simulink model "parrot_gettingstarted"  (R2022a)
settings: Solver=FixedStepAuto  StartTime=0.0  StopTime=100  RelTol=1e-3
InitFcn:
  | load('BusDefinitions.mat')
values from neighbouring files (symbols this model uses):
  all_cov = [0.000210145415622 5.90055533394e-05 -6.5320482463e-06 7.16185822967e-05 0.000233478946029 1.6317851987e-05 7.07877552486e-06 -4.63849255539e-06 -1.33013045343e-05 -0.0012667349074 5.90055533394e-05 0.0112626235932 ... (100 elements, 10x10)]    [cov_data.mat]
  ff = 1.1    [Linearize_Fast.m]
  g = 9.81    [Linearize_Fast.m]    (also in Param_set.m = 9.8)
  ground_alt = 180.2070    (= 180.207)    [Linearize_Fast.m]
  m = 0.068    [Param_set.m]
  Mixer = double(subs(n_lin, [u_vec; a; b; c; d;], [.66708; 0; 0; 0;(1.86e-6);(8.856e-8);(8.856e-8);(9.766e-9)]))    [Linearize_Fast.m]
undefined symbols (not defined in the file or in its folder): codertarget, Discrete, K_PD, K_psi, K_u, K_v, Time
libraries: ctrlSharedLib x5
settings Model: ExtModeTrigDuration=80  Creator=The MathWorks, Inc.  LastModifiedBy=Willi
settings SolverCC: AlgebraicLoopSolver=TrustRegion
settings DataIOCC: ReturnWorkspaceOutputs=off
settings OptimizationCC: PassReuseOutputArgsThreshold=0  MaxStackSize=64
settings DebuggingCC: ParameterTunabilityLossMsg=error  UnconnectedInputMsg=warning  UnconnectedOutputMsg=warning  UnconnectedLineMsg=warning  PregeneratedLibrarySubsystemCodeDiagnostic=none  SFMachineParentedDataDiag=warning  ArithmeticOperatorsInVariantConditions=warning
settings HardwareCC: ProdBitPerPointer=32  ProdBitPerSizeT=32  ProdBitPerPtrDiffT=32  ProdLargestAtomicInteger=Long  ProdWordSize=32  ProdHWDeviceType=ARM Compatible->ARM 9  UseEmbeddedCoderFeatures=off
settings SFSimCC: SimUseLocalCustomCode=off  MATLABDynamicMemAlloc=off  CustomCodeUndefinedFunction=UseInterfaceOnly
settings RTWCC: SystemTargetFile=ert.tlc  HardwareBoard=PARROT Mambo  TemplateMakefile=ert_default_tmf  GenerateReport=on  RTWUseLocalCustomCode=off  Toolchain=Sourcery G++ Lite GNU Toolchain for Drones  BuildConfiguration=Specify  LaunchReport=on
settings CodeAppCC: ForceParamTrailComments=on  OperatorAnnotations=on  StateflowObjectComments=on
settings ERTTargetCC: ERTCustomFileBanners=off  MatFileLogging=on  SupportContinuousTime=on  SupportNonInlinedSFcns=on  RemoveResetFunc=off  ModelStepFunctionPrototypeControlCompliant=off

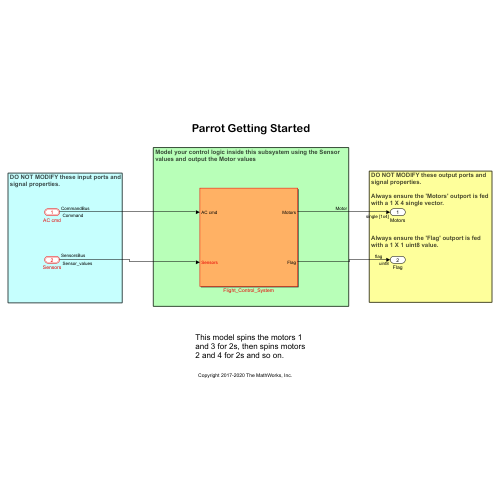
[thumbnail: Simulink's stored preview of the top-level diagram]
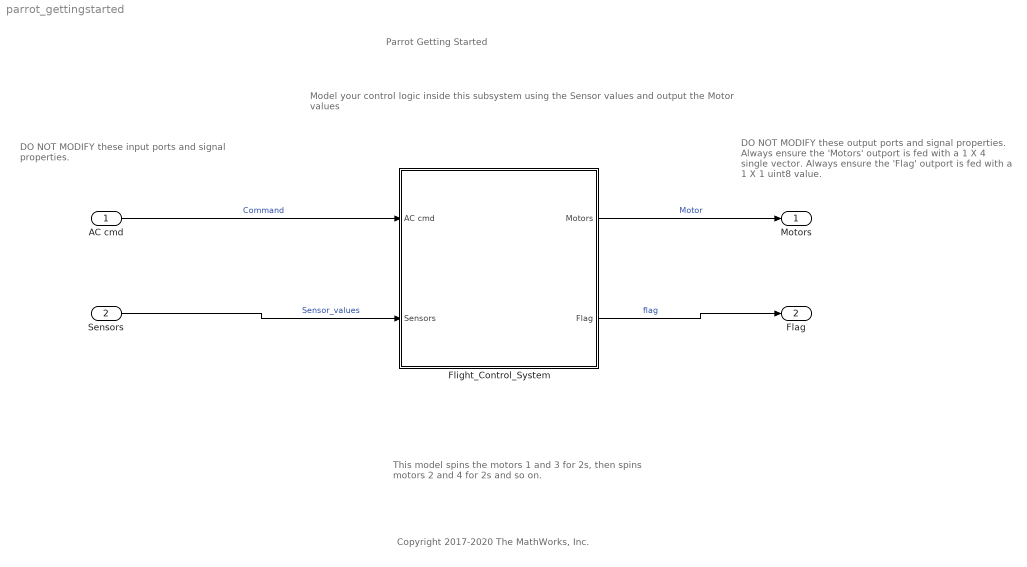
== system parrot_gettingstarted ==
  note: Model your control logic inside this subsystem using the Sensor
      | values and output the Motor values
  note: DO NOT MODIFY these output ports and
      | signal properties.
      |
      | Always ensure the 'Motors' outport is fed
      | with a 1 X 4 single vector.
      |
      |
      |
      |
      | Always ensure the 'Flag' outport is fed
      | with a 1 X 1 uint8 value.
  note: DO NOT MODIFY these input ports and
      | signal properties.
  note: This model spins the motors 1 and 3 for 2s, then spins motors 2 and 4 for 2s and so on.
  note: Copyright 2017-2020 The MathWorks, Inc.
  note: Parrot Getting Started
  AC cmd : Inport  OutDataTypeStr=Bus: CommandBus  BusOutputAsStruct=on
  Sensors : Inport  Port=2  OutDataTypeStr=Bus: SensorsBus  BusOutputAsStruct=on
  Flight_Control_System : Subsystem  InitFcn=codertarget.parrot.internal.fcsSubsystemCallback(gcb);
  Motors : Outport  OutDataTypeStr=single  PortDimensions=[1 4]  VectorParamsAs1DForOutWhenUnconnected=off
  Flag : Outport  Port=2  OutDataTypeStr=uint8  PortDimensions=1  VectorParamsAs1DForOutWhenUnconnected=off
  wires:
  Flight_Control_System/1(Motors) -> Motors/1  "Motor"
  AC cmd/1 -> Flight_Control_System/1(AC cmd)  "Command"
  Sensors/1 -> Flight_Control_System/2(Sensors)  "Sensor_values"
  Flight_Control_System/2(Flag) -> Flag/1  "flag"

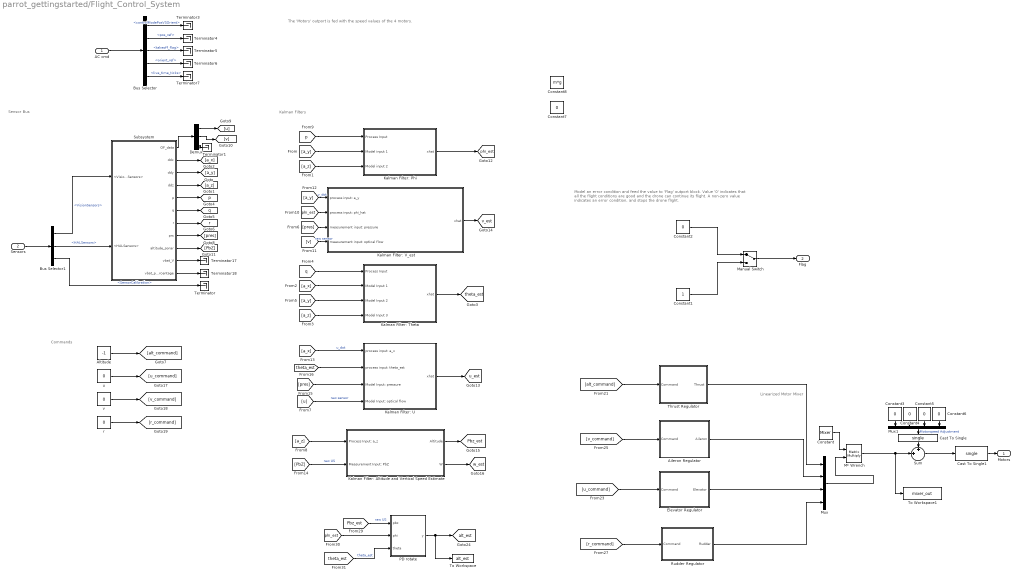
== system parrot_gettingstarted/Flight_Control_System ==
  note: Kalman Filters
  note: Sensor Bus
  note: Linearized Motor Mixer
  note: The 'Motors' outport is fed with the speed values of the 4 motors.
  note: Model an error condition and feed the value to 'Flag' outport block.
      | Value '0' indicates that all the flight conditions are good and the drone
      | can continue its flight.
      | A non-zero value indicates an error condition, and stops the drone
      | flight.
  note: Commands
  AC cmd : Inport
  Sensors : Inport  Port=2
  Aileron Regulator : Subsystem
  Altitude : Constant  Value=-1
  Bus Selector : BusSelector  OutputSignals=controlModePosVSOrient,pos_ref,takeoff_flag,orient_ref,live_time_ticks
  Bus Selector1 : BusSelector  OutputSignals=VisionSensors,HALSensors,SensorCalibration
  Cast To Single : DataTypeConversion  OutDataTypeStr=single  SaturateOnIntegerOverflow=off  RndMeth=Floor
  Cast To Single1 : DataTypeConversion  OutDataTypeStr=single  SaturateOnIntegerOverflow=off  RndMeth=Floor
  Constant : Constant  Value=Mixer
  Constant1 : Constant  OutDataTypeStr=uint8
  Constant2 : Constant  Value=0  OutDataTypeStr=uint8
  Constant{3..7} (5 alike) : Constant  Value=0
  Constant8 : Constant  Value=m*g
  Demux : Demux  Outputs=3
  Elevator Regulator : Subsystem
  Kalman Filter: Altitude and Vertical Speed Estimate : Subsystem
  Kalman Filter: Phi : Subsystem
  Kalman Filter: Theta : Subsystem
  Kalman Filter: U : Subsystem
  Kalman Filter: V_est : Subsystem
  M* Wrench : Product  Multiplication=Matrix(*)
  Manual Switch : ManualSwitch
  Mux : Mux
  Mux1 : Mux
  PD rotate : MATLAB Function  TreatAsAtomicUnit=on
  Rudder Regulator : Subsystem
  Subsystem : Subsystem
  Sum : Sum  Inputs=+|+||
  Terminator{,1,3..7,17..18} (9 alike) : Terminator
  Thrust Regulator : Subsystem
  To Workspace : ToWorkspace  VariableName=alt_est  SaveFormat=Structure With Time  SampleTime=-1
  To Workspace1 : ToWorkspace  VariableName=mixer_out  SaveFormat=Structure With Time  SampleTime=-1
  r : Constant  Value=0
  u : Constant  Value=0
  v : Constant  Value=0
  Motors : Outport  VectorParamsAs1DForOutWhenUnconnected=off
  Flag : Outport  Port=2  VectorParamsAs1DForOutWhenUnconnected=off
  tag scope: Pbz_est=global, alt_est=global, p=global, phi_est=global, q=global, r=global, theta_est=global, u_est=global, v_est=global, w_est=global
  wires:
  AC cmd/1 -> Bus Selector/1
  Bus Selector/1 -> Terminator3/1  "<controlModePosVSOrient>"
  Bus Selector/2 -> Terminator4/1  "<pos_ref>"
  Bus Selector/3 -> Terminator5/1  "<takeoff_flag>"
  Bus Selector/4 -> Terminator6/1  "<orient_ref>"
  Bus Selector/5 -> Terminator7/1  "<live_time_ticks>"
  Manual Switch/1 -> Flag/1
  Constant2/1 -> Manual Switch/1
  Constant1/1 -> Manual Switch/2
  Subsystem/11(vbat_percentage) -> Terminator18/1
  Bus Selector1/3 -> Terminator/1  "<SensorCalibration>"
  Subsystem/8(prs) -> [pres]
  Bus Selector1/2 -> Subsystem/2(<HALSensors>)  "<HALSensors>"
  Bus Selector1/1 -> Subsystem/1(<VisionSensors>)  "<VisionSensors>"
  Subsystem/1(OF_data) -> Demux/1
  Subsystem/4(ddz) -> [a_z]
  Subsystem/3(ddy) -> [a_y]
  Subsystem/9(altitude_sonar) -> [PbZ]
  Subsystem/10(vbat_V) -> Terminator17/1
  Subsystem/2(ddx) -> [a_x]
  Sensors/1 -> Bus Selector1/1
  Sum/1 -> Cast To Single1/1
  Mux1/1 -> Cast To Single/1  "Motorspeed Adjustment"
  Cast To Single/1 -> Sum/1
  Constant6/1 -> Mux1/4
  Constant5/1 -> Mux1/3
  Constant3/1 -> Mux1/1
  Constant4/1 -> Mux1/2
  Constant/1 -> M* Wrench/1
  Demux/1 -> [u]
  Demux/2 -> [v]
  Demux/3 -> Terminator1/1
  Subsystem/5(p) -> [p]
  Subsystem/6(q) -> [q]
  Subsystem/7(r) -> [r]
  [a_z] -> Kalman Filter: Phi/3(Model input 2)
  [a_y] -> Kalman Filter: Phi/2(Model input 1)
  Kalman Filter: Phi/1(xhat) -> [phi_est]
  [p] -> Kalman Filter: Phi/1(Process Input)
  [q] -> Kalman Filter: Theta/1(Process Input)
  Kalman Filter: Theta/1(xhat) -> [theta_est]
  [a_z] -> Kalman Filter: Theta/4(Model Input 3)
  [a_x] -> Kalman Filter: Theta/2(Model Input 1)
  [a_y] -> Kalman Filter: Theta/3(Model Input 2)
  [theta_est] -> Kalman Filter: U/2(process input: theta_est)
  [u] -> Kalman Filter: U/4(Model Input: optical flow)  "raw sensor"
  [a_x] -> Kalman Filter: U/1(process input: a_x)  "u_dot"
  Kalman Filter: U/1(xhat) -> [u_est]
  [pres] -> Kalman Filter: U/3(Model Input: pressure)
  [a_z] -> Kalman Filter: Altitude and Vertical Speed Estimate/1("Process Input: a_z ")
  Kalman Filter: Altitude and Vertical Speed Estimate/1(Altitude) -> [Pbz_est]
  [PbZ] -> Kalman Filter: Altitude and Vertical Speed Estimate/2(Measurement Input: PbZ)  "raw US"
  Kalman Filter: Altitude and Vertical Speed Estimate/2(W) -> [w_est]
  [a_y] -> Kalman Filter: V_est/1("process input: a_y   ")  "v_dot"
  [pres] -> Kalman Filter: V_est/3(measurement input: pressure)
  [v] -> Kalman Filter: V_est/4(measurement input: optical flow)  "raw sensor"
  Kalman Filter: V_est/1(xhat) -> [v_est]
  [phi_est] -> Kalman Filter: V_est/2("process input: phi_hat ")
  [theta_est] -> PD rotate/3(theta)  "theta_est"
  PD rotate/1(y) -> To Workspace/1, [alt_est]
  [Pbz_est] -> PD rotate/1(pbz)  "raw US"
  [phi_est] -> PD rotate/2(phi)
  r/1 -> [r_command]
  v/1 -> [v_command]
  u/1 -> [u_command]
  Altitude/1 -> [alt_command]
  [alt_command] -> Thrust Regulator/1(Command)
  Mux/1 -> M* Wrench/2
  Cast To Single1/1 -> Motors/1
  M* Wrench/1 -> Sum/2, To Workspace1/1
  [r_command] -> Rudder Regulator/1(Command)
  [u_command] -> Elevator Regulator/1(Command)
  [v_command] -> Aileron Regulator/1(Command)
  Rudder Regulator/1(Rudder) -> Mux/4
  Thrust Regulator/1(Thrust) -> Mux/1
  Elevator Regulator/1(Elevator) -> Mux/3
  Aileron Regulator/1(Aileron) -> Mux/2

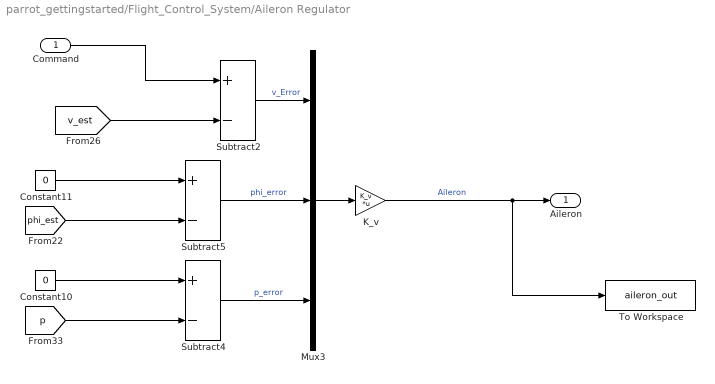
== system parrot_gettingstarted/Flight_Control_System/Aileron Regulator ==
  Command : Inport
  Constant10 : Constant  Value=0
  Constant11 : Constant  Value=0
  K_v : Gain  Gain=K_v  Multiplication=Matrix(K*u)
  Mux3 : Mux  Inputs=3
  Subtract2 : Sum  Inputs=+-
  Subtract4 : Sum  Inputs=+-
  Subtract5 : Sum  Inputs=+-
  To Workspace : ToWorkspace  VariableName=aileron_out  SaveFormat=Timeseries  SampleTime=-1
  Aileron : Outport
  wires:
  [p] -> Subtract4/2
  [v_est] -> Subtract2/2
  Constant11/1 -> Subtract5/1
  [phi_est] -> Subtract5/2
  Subtract5/1 -> Mux3/2  "phi_error"
  Subtract2/1 -> Mux3/1  "v_Error"
  Mux3/1 -> K_v/1
  Subtract4/1 -> Mux3/3  "p_error"
  Constant10/1 -> Subtract4/1
  K_v/1 -> To Workspace/1, Aileron/1  "Aileron"
  Command/1 -> Subtract2/1

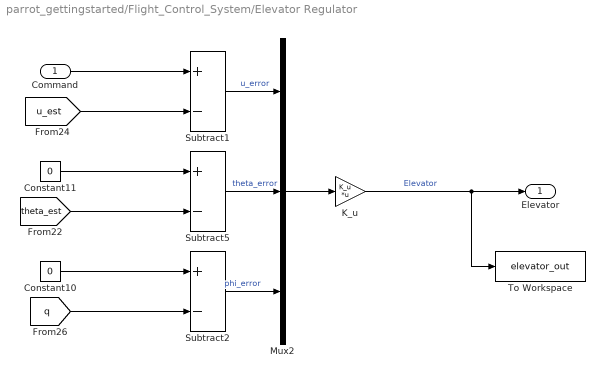
== system parrot_gettingstarted/Flight_Control_System/Elevator Regulator ==
  Command : Inport
  Constant10 : Constant  Value=0
  Constant11 : Constant  Value=0
  K_u : Gain  Gain=K_u  Multiplication=Matrix(K*u)
  Mux2 : Mux  Inputs=3
  Subtract1 : Sum  Inputs=+-
  Subtract2 : Sum  Inputs=+-
  Subtract5 : Sum  Inputs=+-
  To Workspace : ToWorkspace  VariableName=elevator_out  SaveFormat=Timeseries  SampleTime=-1
  Elevator : Outport
  wires:
  [theta_est] -> Subtract5/2
  [u_est] -> Subtract1/2
  Constant10/1 -> Subtract2/1
  Constant11/1 -> Subtract5/1
  Subtract5/1 -> Mux2/2  "theta_error"
  Subtract1/1 -> Mux2/1  "u_error"
  Subtract2/1 -> Mux2/3  "phi_error"
  Mux2/1 -> K_u/1
  [q] -> Subtract2/2
  K_u/1 -> To Workspace/1, Elevator/1  "Elevator"
  Command/1 -> Subtract1/1

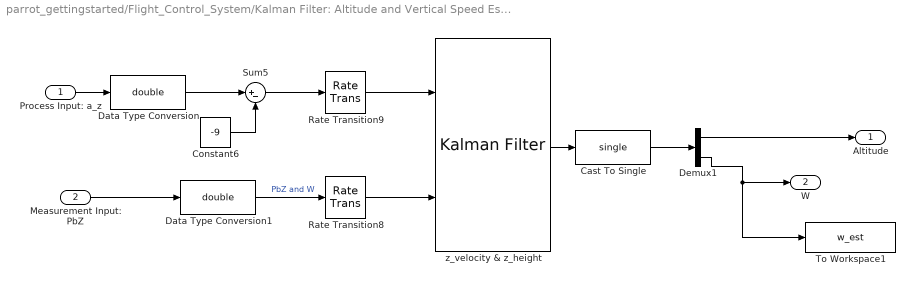
== system parrot_gettingstarted/Flight_Control_System/Kalman Filter: Altitude and Vertical Speed Estimate ==
  "Process Input: a_z " : Inport
  Measurement Input: PbZ : Inport  Port=2
  Cast To Single : DataTypeConversion  OutDataTypeStr=single  SaturateOnIntegerOverflow=off  RndMeth=Floor
  Constant6 : Constant  Value=-9
  Data Type Conversion : DataTypeConversion  OutDataTypeStr=double  SaturateOnIntegerOverflow=off  RndMeth=Floor
  Data Type Conversion1 : DataTypeConversion  OutDataTypeStr=double  SaturateOnIntegerOverflow=off  RndMeth=Floor
  Demux1 : Demux  Outputs=2
  Rate Transition8 : RateTransition  OutPortSampleTime=1/200
  Rate Transition9 : RateTransition  OutPortSampleTime=1/200
  Sum5 : Sum  Inputs=|+-
  To Workspace1 : ToWorkspace  VariableName=w_est  SaveFormat=Structure With Time  SampleTime=-1
  z_velocity & z_height : ctrlSharedLib/Kalman Filter  TimeDomain=Discrete-Time  UseCurrentEstimator=on  ModelSource=Individual A, B, C, D matrices  ModelSourceVariable=ss(0.95,1,1,0,1)  A=[1 1/200;0 1]  B=[0; 1/200]  C=[1 0]  D=0  NumberOfStates=1  NumberOfInputs=1  NumberOfOutputs=1  InitialEstimateSource=Dialog  X0=0  P0=10  UseK=off  UseGH=off  NumberOfProcessNoiseInputs=1  G=1  TimeInvariantG=on  H=0  TimeInvariantH=on  Q=all_cov(7,7)/1000  TimeInvariantQ=on  R=all_cov(1,1)*50  TimeInvariantR=on  N=0  TimeInvariantN=on  AddInputPort=on  AddEnablePort=off  OutputEstimatedY=off  OutputP=off  Ts=-1
  Altitude : Outport
  W : Outport  Port=2
  wires:
  Data Type Conversion1/1 -> Rate Transition8/1  "PbZ and W"
  Constant6/1 -> Sum5/2
  Demux1/1 -> Altitude/1
  z_velocity & z_height/1 -> Cast To Single/1
  Sum5/1 -> Rate Transition9/1
  Data Type Conversion/1 -> Sum5/1
  Rate Transition9/1 -> z_velocity & z_height/1
  Rate Transition8/1 -> z_velocity & z_height/2
  Measurement Input: PbZ/1 -> Data Type Conversion1/1
  Demux1/2 -> W/1, To Workspace1/1
  "Process Input: a_z "/1 -> Data Type Conversion/1
  Cast To Single/1 -> Demux1/1

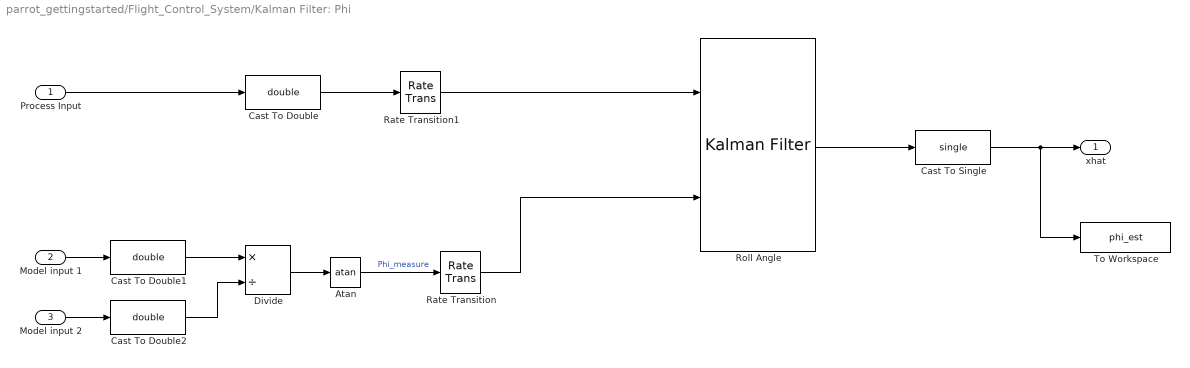
== system parrot_gettingstarted/Flight_Control_System/Kalman Filter: Phi ==
  Process Input : Inport
  Model input 1 : Inport  Port=2
  Model input 2 : Inport  Port=3
  Atan : Trigonometry  Operator=atan
  Cast To Double : DataTypeConversion  OutDataTypeStr=double  SaturateOnIntegerOverflow=off  RndMeth=Floor
  Cast To Double1 : DataTypeConversion  OutDataTypeStr=double  SaturateOnIntegerOverflow=off  RndMeth=Floor
  Cast To Double2 : DataTypeConversion  OutDataTypeStr=double  SaturateOnIntegerOverflow=off  RndMeth=Floor
  Cast To Single : DataTypeConversion  OutMax=1  OutDataTypeStr=single  SaturateOnIntegerOverflow=off  RndMeth=Floor
  Divide : Product  Inputs=*/
  Rate Transition : RateTransition  OutPortSampleTime=1/200
  Rate Transition1 : RateTransition  OutPortSampleTime=1/200
  Roll Angle : ctrlSharedLib/Kalman Filter  TimeDomain=Discrete-Time  UseCurrentEstimator=on  ModelSource=Individual A, B, C, D matrices  ModelSourceVariable=ss(0.95,1,1,0,1)  A=[1]  B=[1/200]  C=[1]  D=0  NumberOfStates=1  NumberOfInputs=1  NumberOfOutputs=1  InitialEstimateSource=Dialog  X0=0  P0=10  UseK=off  UseGH=off  NumberOfProcessNoiseInputs=1  G=1  TimeInvariantG=on  H=0  TimeInvariantH=on  Q=.0133/200  TimeInvariantQ=on  R=.0101  TimeInvariantR=on  N=0  TimeInvariantN=on  AddInputPort=on  AddEnablePort=off  OutputEstimatedY=off  OutputP=off  Ts=-1
  To Workspace : ToWorkspace  VariableName=phi_est  SaveFormat=Structure With Time  SampleTime=-1
  xhat : Outport
  wires:
  Divide/1 -> Atan/1
  Atan/1 -> Rate Transition/1  "Phi_measure"
  Process Input/1 -> Cast To Double/1
  Rate Transition/1 -> Roll Angle/2
  Rate Transition1/1 -> Roll Angle/1
  Cast To Double/1 -> Rate Transition1/1
  Cast To Double1/1 -> Divide/1
  Model input 1/1 -> Cast To Double1/1
  Model input 2/1 -> Cast To Double2/1
  Cast To Double2/1 -> Divide/2
  Cast To Single/1 -> To Workspace/1, xhat/1
  Roll Angle/1 -> Cast To Single/1

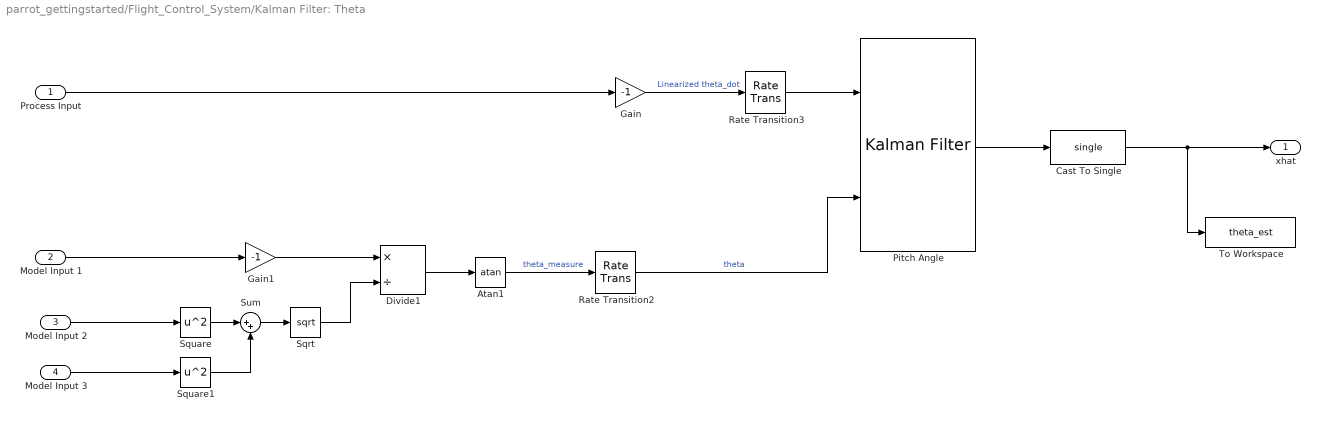
== system parrot_gettingstarted/Flight_Control_System/Kalman Filter: Theta ==
  Process Input : Inport
  Model Input 1 : Inport  Port=2
  Model Input 2 : Inport  Port=3
  Model Input 3 : Inport  Port=4
  Atan1 : Trigonometry  Operator=atan
  Cast To Single : DataTypeConversion  OutDataTypeStr=single  SaturateOnIntegerOverflow=off  RndMeth=Floor
  Divide1 : Product  Inputs=*/
  Gain : Gain  Gain=-1
  Gain1 : Gain  Gain=-1
  Pitch Angle : ctrlSharedLib/Kalman Filter  TimeDomain=Discrete-Time  UseCurrentEstimator=on  ModelSource=Individual A, B, C, D matrices  ModelSourceVariable=ss(0.95,1,1,0,1)  A=[1]  B=[1/200]  C=[1]  D=0  NumberOfStates=1  NumberOfInputs=1  NumberOfOutputs=1  InitialEstimateSource=Dialog  X0=0  P0=10  UseK=off  UseGH=off  NumberOfProcessNoiseInputs=1  G=1  TimeInvariantG=on  H=0  TimeInvariantH=on  Q=.0085/1000  TimeInvariantQ=on  R=.0066/10  TimeInvariantR=on  N=0  TimeInvariantN=on  AddInputPort=on  AddEnablePort=off  OutputEstimatedY=off  OutputP=off  Ts=-1
  Rate Transition2 : RateTransition  OutPortSampleTime=1/200
  Rate Transition3 : RateTransition  OutPortSampleTime=1/200
  Sqrt : Sqrt
  Square : Math  Operator=square
  Square1 : Math  Operator=square
  Sum : Sum  Inputs=|++
  To Workspace : ToWorkspace  VariableName=theta_est  SaveFormat=Structure With Time  SampleTime=-1
  xhat : Outport
  wires:
  Gain1/1 -> Divide1/1
  Divide1/1 -> Atan1/1
  Model Input 2/1 -> Square/1
  Rate Transition3/1 -> Pitch Angle/1
  Sum/1 -> Sqrt/1
  Square/1 -> Sum/1
  Square1/1 -> Sum/2
  Atan1/1 -> Rate Transition2/1  "theta_measure"
  Sqrt/1 -> Divide1/2
  Rate Transition2/1 -> Pitch Angle/2  "theta"
  Gain/1 -> Rate Transition3/1  "Linearized theta_dot"
  Process Input/1 -> Gain/1
  Model Input 1/1 -> Gain1/1
  Model Input 3/1 -> Square1/1
  Cast To Single/1 -> xhat/1, To Workspace/1
  Pitch Angle/1 -> Cast To Single/1

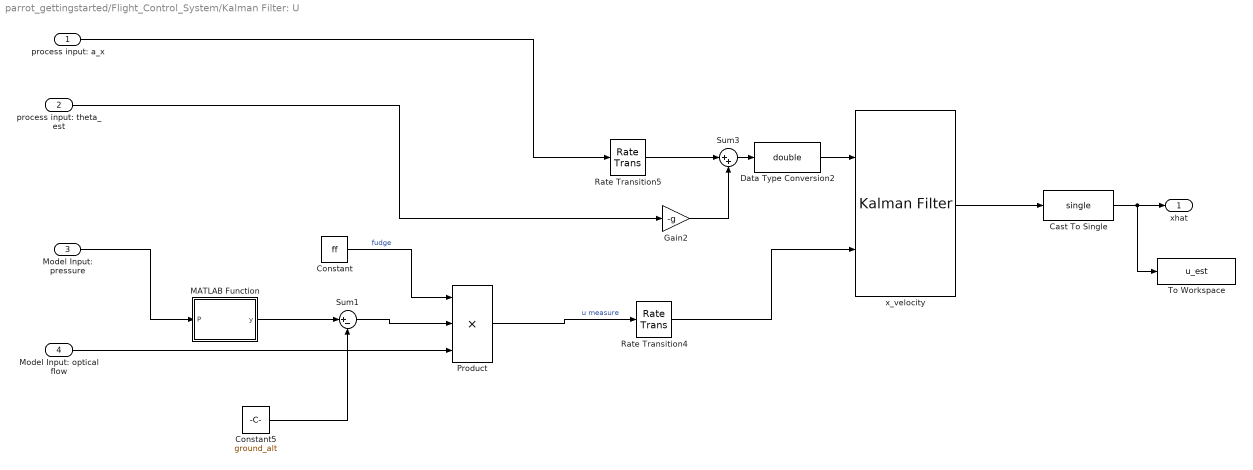
== system parrot_gettingstarted/Flight_Control_System/Kalman Filter: U ==
  process input: a_x : Inport
  process input: theta_est : Inport  Port=2
  Model Input: pressure : Inport  Port=3
  Model Input: optical flow : Inport  Port=4
  Cast To Single : DataTypeConversion  OutDataTypeStr=single  SaturateOnIntegerOverflow=off  RndMeth=Floor
  Constant : Constant  Value=ff
  Constant5 : Constant  Value=ground_alt
  Data Type Conversion2 : DataTypeConversion  OutDataTypeStr=double  SaturateOnIntegerOverflow=off  RndMeth=Floor
  Gain2 : Gain  Gain=-g
  MATLAB Function : MATLAB Function  TreatAsAtomicUnit=on
  Product : Product  Inputs=3
  Rate Transition4 : RateTransition  OutPortSampleTime=1/200
  Rate Transition5 : RateTransition  OutPortSampleTime=1/200
  Sum1 : Sum  Inputs=|+-
  Sum3 : Sum  Inputs=|++
  To Workspace : ToWorkspace  VariableName=u_est  SaveFormat=Structure With Time  SampleTime=-1
  x_velocity : ctrlSharedLib/Kalman Filter  TimeDomain=Discrete-Time  UseCurrentEstimator=on  ModelSource=Individual A, B, C, D matrices  ModelSourceVariable=ss(0.95,1,1,0,1)  A=[1]  B=[1/200]  C=[1]  D=0  NumberOfStates=1  NumberOfInputs=1  NumberOfOutputs=1  InitialEstimateSource=Dialog  X0=0  P0=10  UseK=off  UseGH=off  NumberOfProcessNoiseInputs=1  G=1  TimeInvariantG=on  H=0  TimeInvariantH=on  Q=.0059/200  TimeInvariantQ=on  R=all_cov(10,8)*20  TimeInvariantR=on  N=0  TimeInvariantN=on  AddInputPort=on  AddEnablePort=off  OutputEstimatedY=off  OutputP=off  Ts=-1
  xhat : Outport
  wires:
  process input: theta_est/1 -> Gain2/1
  MATLAB Function/1(y) -> Sum1/1
  Gain2/1 -> Sum3/2
  Product/1 -> Rate Transition4/1  "u measure"
  Rate Transition4/1 -> x_velocity/2
  process input: a_x/1 -> Rate Transition5/1
  Rate Transition5/1 -> Sum3/1
  Sum1/1 -> Product/2
  Data Type Conversion2/1 -> x_velocity/1
  Constant/1 -> Product/1  "fudge"
  Sum3/1 -> Data Type Conversion2/1
  Constant5/1 -> Sum1/2
  Model Input: pressure/1 -> MATLAB Function/1(P)
  Model Input: optical flow/1 -> Product/3
  Cast To Single/1 -> To Workspace/1, xhat/1
  x_velocity/1 -> Cast To Single/1

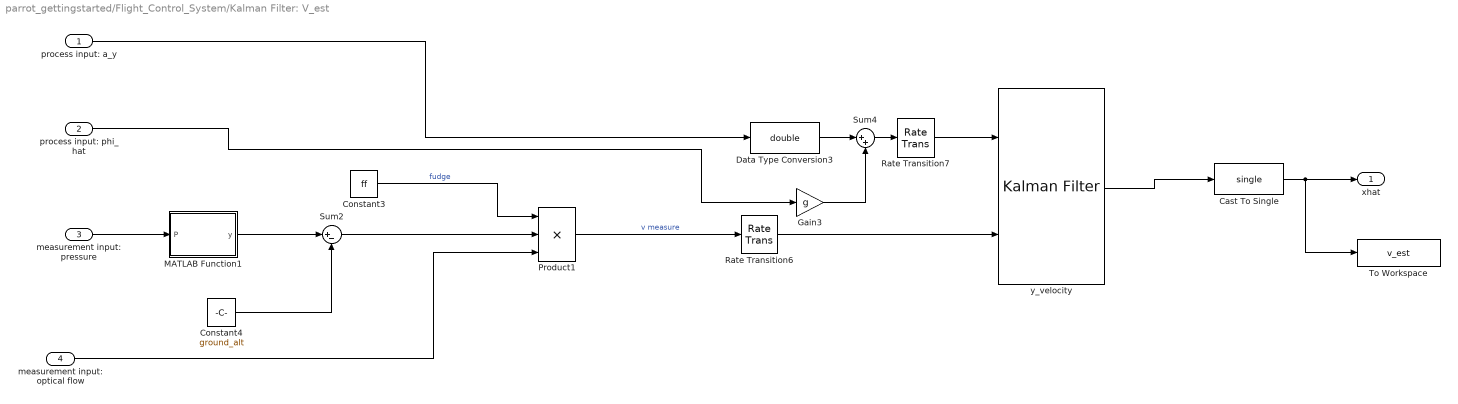
== system parrot_gettingstarted/Flight_Control_System/Kalman Filter: V_est ==
  "process input: a_y   " : Inport
  "process input: phi_hat " : Inport  Port=2
  measurement input: pressure : Inport  Port=3
  measurement input: optical flow : Inport  Port=4
  Cast To Single : DataTypeConversion  OutDataTypeStr=single  SaturateOnIntegerOverflow=off  RndMeth=Floor
  Constant3 : Constant  Value=ff
  Constant4 : Constant  Value=ground_alt
  Data Type Conversion3 : DataTypeConversion  OutDataTypeStr=double  SaturateOnIntegerOverflow=off  RndMeth=Floor
  Gain3 : Gain  Gain=g
  MATLAB Function1 : MATLAB Function  TreatAsAtomicUnit=on
  Product1 : Product  Inputs=3
  Rate Transition6 : RateTransition  OutPortSampleTime=1/200
  Rate Transition7 : RateTransition  OutPortSampleTime=1/200
  Sum2 : Sum  Inputs=|+-
  Sum4 : Sum  Inputs=|++
  To Workspace : ToWorkspace  VariableName=v_est  SaveFormat=Structure With Time  SampleTime=-1
  y_velocity : ctrlSharedLib/Kalman Filter  TimeDomain=Discrete-Time  UseCurrentEstimator=on  ModelSource=Individual A, B, C, D matrices  ModelSourceVariable=ss(0.95,1,1,0,1)  A=[1]  B=[1/200]  C=[1]  D=0  NumberOfStates=1  NumberOfInputs=1  NumberOfOutputs=1  InitialEstimateSource=Dialog  X0=0  P0=10  UseK=off  UseGH=off  NumberOfProcessNoiseInputs=1  G=1  TimeInvariantG=on  H=0  TimeInvariantH=on  Q=.0087/200  TimeInvariantQ=on  R=2.5  TimeInvariantR=on  N=0  TimeInvariantN=on  AddInputPort=on  AddEnablePort=off  OutputEstimatedY=off  OutputP=off  Ts=-1
  xhat : Outport
  wires:
  MATLAB Function1/1(y) -> Sum2/1
  Gain3/1 -> Sum4/2
  Sum2/1 -> Product1/2
  measurement input: optical flow/1 -> Product1/3
  Constant4/1 -> Sum2/2
  Product1/1 -> Rate Transition6/1  "v measure"
  Rate Transition6/1 -> y_velocity/2
  Sum4/1 -> Rate Transition7/1
  Constant3/1 -> Product1/1  "fudge"
  Rate Transition7/1 -> y_velocity/1
  Data Type Conversion3/1 -> Sum4/1
  "process input: phi_hat "/1 -> Gain3/1
  measurement input: pressure/1 -> MATLAB Function1/1(P)
  "process input: a_y   "/1 -> Data Type Conversion3/1
  Cast To Single/1 -> To Workspace/1, xhat/1
  y_velocity/1 -> Cast To Single/1

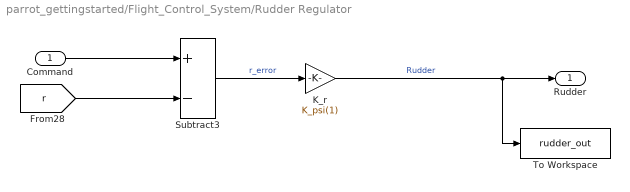
== system parrot_gettingstarted/Flight_Control_System/Rudder Regulator ==
  Command : Inport
  K_r : Gain  Gain=K_psi(1)
  Subtract3 : Sum  Inputs=+-
  To Workspace : ToWorkspace  VariableName=rudder_out  SaveFormat=Timeseries  SampleTime=-1
  Rudder : Outport
  wires:
  Subtract3/1 -> K_r/1  "r_error"
  K_r/1 -> To Workspace/1, Rudder/1  "Rudder"
  [r] -> Subtract3/2
  Command/1 -> Subtract3/1

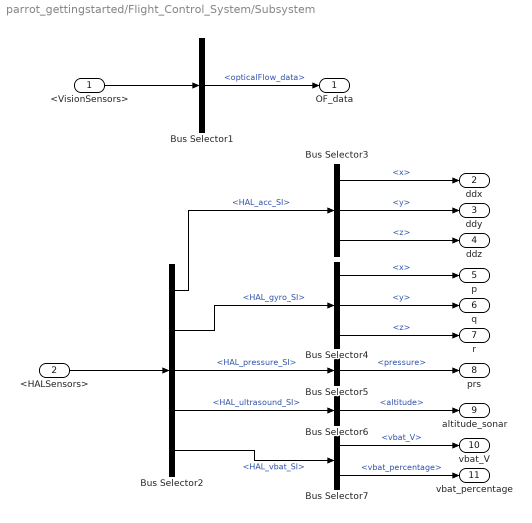
== system parrot_gettingstarted/Flight_Control_System/Subsystem ==
  <VisionSensors> : Inport
  <HALSensors> : Inport  Port=2
  Bus Selector1 : BusSelector  OutputSignals=opticalFlow_data
  Bus Selector2 : BusSelector  OutputSignals=HAL_acc_SI,HAL_gyro_SI,HAL_pressure_SI,HAL_ultrasound_SI,HAL_vbat_SI
  Bus Selector3 : BusSelector  OutputSignals=x,y,z
  Bus Selector4 : BusSelector  OutputSignals=x,y,z
  Bus Selector5 : BusSelector  OutputSignals=pressure
  Bus Selector6 : BusSelector  OutputSignals=altitude
  Bus Selector7 : BusSelector  OutputSignals=vbat_V,vbat_percentage
  OF_data : Outport  VectorParamsAs1DForOutWhenUnconnected=off
  ddx : Outport  Port=2  VectorParamsAs1DForOutWhenUnconnected=off
  ddy : Outport  Port=3  VectorParamsAs1DForOutWhenUnconnected=off
  ddz : Outport  Port=4  VectorParamsAs1DForOutWhenUnconnected=off
  p : Outport  Port=5  VectorParamsAs1DForOutWhenUnconnected=off
  q : Outport  Port=6  VectorParamsAs1DForOutWhenUnconnected=off
  r : Outport  Port=7  VectorParamsAs1DForOutWhenUnconnected=off
  prs : Outport  Port=8  VectorParamsAs1DForOutWhenUnconnected=off
  altitude_sonar : Outport  Port=9  VectorParamsAs1DForOutWhenUnconnected=off
  vbat_V : Outport  Port=10  VectorParamsAs1DForOutWhenUnconnected=off
  vbat_percentage : Outport  Port=11  VectorParamsAs1DForOutWhenUnconnected=off
  wires:
  <VisionSensors>/1 -> Bus Selector1/1
  <HALSensors>/1 -> Bus Selector2/1
  Bus Selector1/1 -> OF_data/1  "<opticalFlow_data>"
  Bus Selector2/1 -> Bus Selector3/1  "<HAL_acc_SI>"
  Bus Selector2/2 -> Bus Selector4/1  "<HAL_gyro_SI>"
  Bus Selector2/3 -> Bus Selector5/1  "<HAL_pressure_SI>"
  Bus Selector2/4 -> Bus Selector6/1  "<HAL_ultrasound_SI>"
  Bus Selector2/5 -> Bus Selector7/1  "<HAL_vbat_SI>"
  Bus Selector3/1 -> ddx/1  "<x>"
  Bus Selector3/2 -> ddy/1  "<y>"
  Bus Selector3/3 -> ddz/1  "<z>"
  Bus Selector4/2 -> q/1  "<y>"
  Bus Selector4/1 -> p/1  "<x>"
  Bus Selector4/3 -> r/1  "<z>"
  Bus Selector5/1 -> prs/1  "<pressure>"
  Bus Selector6/1 -> altitude_sonar/1  "<altitude>"
  Bus Selector7/1 -> vbat_V/1  "<vbat_V>"
  Bus Selector7/2 -> vbat_percentage/1  "<vbat_percentage>"

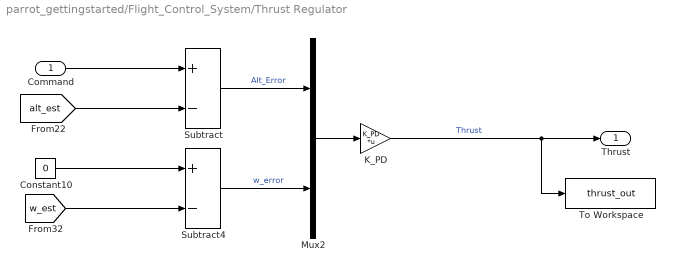
== system parrot_gettingstarted/Flight_Control_System/Thrust Regulator ==
  Command : Inport
  Constant10 : Constant  Value=0
  K_PD : Gain  Gain=K_PD  Multiplication=Matrix(K*u)
  Mux2 : Mux  Inputs=2
  Subtract : Sum  Inputs=+-
  Subtract4 : Sum  Inputs=+-
  To Workspace : ToWorkspace  VariableName=thrust_out  SaveFormat=Structure With Time  SampleTime=-1
  Thrust : Outport
  wires:
  Subtract4/1 -> Mux2/2  "w_error"
  [w_est] -> Subtract4/2
  [alt_est] -> Subtract/2
  Subtract/1 -> Mux2/1  "Alt_Error"
  K_PD/1 -> To Workspace/1, Thrust/1  "Thrust"
  Command/1 -> Subtract/1
  Constant10/1 -> Subtract4/1
  Mux2/1 -> K_PD/1

== matlab function parrot_gettingstarted/Flight_Control_System/Kalman Filter: U/MATLAB Function ==
  data: P input; y output
function y = z_pres(P)
g = 9.8; % acceleration due to gravity m/s^2
M = 0.0289644; % molar mass of air in kg/mol
R = 8.31432; % universal gas constant Nm/mol/k
p0 = 101325; % Pa standard pressure

T =288.15;  % Assumed temperature in kelvin
K =-g*M/R/T;
z_hypsometric = 1/K*log(P/p0);
y = z_hypsometric;

== matlab function parrot_gettingstarted/Flight_Control_System/PD rotate ==
  data: pbz input; y output; phi input; theta input
function y = rotate_BE(pbz, phi, theta)
roll_BE = [1 0 0; 0 cos(phi) sin(phi); 0 -sin(phi) cos(phi)]';
pitch_BE = [cos(theta) 0 -sin(theta); 0 1 0; sin(theta) 0 cos(theta);]';
%yaw_BE = simplify(inv([cos(psi) sin(psi) 0; -sin(psi) cos(psi) 0; 0 0 1;]));
rotater = roll_BE*pitch_BE*pbz;
y = rotater(3);

== matlab function parrot_gettingstarted/Flight_Control_System/Kalman Filter: V_est/MATLAB Function1 ==
  data: P input; y output
function y = z_pres(P)
g = 9.8; % acceleration due to gravity m/s^2
M = 0.0289644; % molar mass of air in kg/mol
R = 8.31432; % universal gas constant Nm/mol/k
p0 = 101325; % Pa standard pressure

T =288.15;  % Assumed temperature in kelvin
K =-g*M/R/T;
z_hypsometric = 1/K*log(P/p0);
y = z_hypsometric;
